simulink model "Model_3c_2015a"  (R2015a)
settings: Solver=ode45  StartTime=0.0  StopTime=40  RelTol=1e-3
undefined symbols (not defined in the file): c1, c2, K1, K2, K3, Ts, wave
settings Model: CovModelRefEnable=off  Creator=s3blanch  LastModifiedBy=s3blanch
settings DataIOCC: SaveFormat=StructureWithTime
settings HardwareCC: ProdBitPerPointer=64  ProdLargestAtomicFloat=Float  ProdIntDivRoundTo=Zero  ProdEndianess=LittleEndian  ProdHWDeviceType=Specified
settings GRTTargetCC: GeneratePreprocessorConditionals=Use local settings

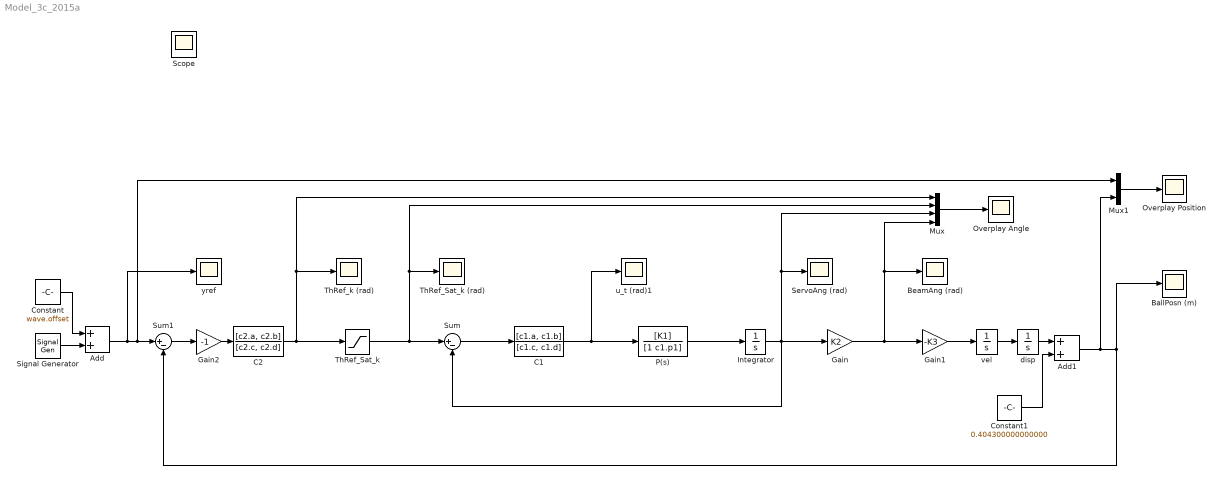
== system Model_3c_2015a ==
  " BeamAng (rad)" : Scope
      settings: TimeRange=auto  MaxDataPoints=5000  SaveName=BeamAng  YMin=-0.03886  YMax=0.03886  SampleTime=-1  DataFormat=Array
  Add : Sum
  Add1 : Sum
  BallPosn (m) : Scope
      settings: TimeRange=auto  MaxDataPoints=5000  SaveName=BallPosn  YMin=0  YMax=0.5  SampleTime=-1  DataFormat=Array
  C1 : DiscreteTransferFcn  Numerator=[c1.a, c1.b]  Denominator=[c1.c, c1.d]  SampleTime=Ts
  C2 : DiscreteTransferFcn  Numerator=[c2.a, c2.b]  Denominator=[c2.c, c2.d]  SampleTime=Ts
  Constant : Constant  Value=wave.offset
  Constant1 : Constant  Value=0.404300000000000
  Gain : Gain  Gain=K2
  Gain1 : Gain  Gain=-K3
  Gain2 : Gain  Gain=-1
  Integrator : Integrator
  Mux : Mux
  Mux1 : Mux  Inputs=2
  Overplay Angle : Scope
      settings: TimeRange=25  MaxDataPoints=5000  SaveToWorkspace=off  YMin=-1.05154  YMax=1.20456  SampleTime=-1  DataFormat=Array
  Overplay Position : Scope
      settings: TimeRange=25  MaxDataPoints=5000  SaveToWorkspace=off  SaveName=ScopeData  YMin=0.10696  YMax=0.43734  SampleTime=-1  DataFormat=Array
  P(s) : TransferFcn  Numerator=[K1]  Denominator=[1 c1.p1]
  ServoAng (rad) : Scope
      settings: TimeRange=auto  MaxDataPoints=5000  SaveName=ServoAng  YMin=-0.63804  YMax=0.63804  SampleTime=-1  DataFormat=Array
  Signal Generator : SignalGenerator  WaveForm=square  Amplitude=-wave.amp  Frequency=0.05
  Sum : Sum  Inputs=|+-
  Sum1 : Sum  Inputs=|+-
  ThRef_Sat_k : Saturate  UpperLimit=0.7  LowerLimit=-0.7
  ThRef_Sat_k (rad) : Scope
      settings: TimeRange=auto  MaxDataPoints=5000  SaveName=ThRef  YMin=-0.875  YMax=0.875  SampleTime=-1  DataFormat=Array
  ThRef_k (rad) : Scope
      settings: TimeRange=auto  MaxDataPoints=5000  SaveName=ref  YMin=-7.58392  YMax=7.58391  SampleTime=-1  DataFormat=Array
  disp : Integrator
  u_t (rad)1 : Scope
      settings: TimeRange=auto  MaxDataPoints=5000  SaveName=u  YMin=-3.50155  YMax=2.92902  SampleTime=-1  DataFormat=Array
  vel : Integrator
  yref : Scope
      settings: TimeRange=auto  MaxDataPoints=5000  SaveName=yref  YMin=0.1275  YMax=0.2525  SampleTime=-1  DataFormat=Array
  Scope : Scope
      settings: TimeRange=auto  MaxDataPoints=5000  SaveToWorkspace=off  YMin=-0.70238  YMax=0.70238  SampleTime=-1
  wires:
  P(s)/1 -> Integrator/1
  Integrator/1 -> Gain/1, Sum/2, Mux/3, ServoAng (rad)/1
  Mux/1 -> Overplay Angle/1
  Sum/1 -> C1/1
  C1/1 -> P(s)/1, u_t (rad)1/1
  Gain1/1 -> vel/1
  vel/1 -> disp/1
  C2/1 -> Mux/1, ThRef_k (rad)/1, ThRef_Sat_k/1
  Mux1/1 -> Overplay Position/1
  Signal Generator/1 -> Add/2
  Constant/1 -> Add/1
  Add/1 -> Mux1/1, Sum1/1, yref/1
  Gain/1 -> Gain1/1, " BeamAng (rad)"/1, Mux/4
  ThRef_Sat_k/1 -> Sum/1, Mux/2, ThRef_Sat_k (rad)/1
  disp/1 -> Add1/1
  Add1/1 -> Mux1/2, Sum1/2, BallPosn (m)/1
  Constant1/1 -> Add1/2
  Sum1/1 -> Gain2/1
  Gain2/1 -> C2/1
